simulink model "MPC_framework"  (Simulink 6.4)
settings: Solver=FixedStepDiscrete  StartTime=0.0  StopTime=10.0  FixedStep=0.01  RelTol=1e-3
PreLoadFcn:
  | RTWConfigurationCB('preloadfcn', bdroot);
InitFcn:
  | % START RTW CONFIGURATION CODE %
  | RTWConfigurationCB('rtw_target_initfcn',gcs);
  | % END RTW CONFIGURATION CODE %
undefined symbols (not defined in the file): a1, a2, DA_max_saturation, DA_min_saturation, DiscIntNeverNeededParam, fundamental_sample_time, incntr_half_val, init_1_message, init_2_message, init_ack_async_message, init_ack_sync_message, motor_negative_value_seg_1, motor_negative_value_seg_2, motor_positive_value_seg_1, motor_positive_value_seg_2, motor_stopped_value, ticks_per_trajectory_time, trajectory_time
libraries: canblocks x16, mpc555toucan x16, simulink x8, mpc555drivers x1
(part 1 of 2)
CloseFcn:
  | rtwprivate ssgencode ModelCloseRequest MPC_framework
settings Model: LastModifiedBy=Developer  ProdHWDeviceType=Motorola PowerPC
settings OptimizationCC: OptimizeModelRefInitCode=on  LifeSpan=1
settings HardwareCC: ProdIntDivRoundTo=Zero  ProdEndianess=BigEndian  ProdHWDeviceType=Motorola PowerPC
settings RTWCC: SystemTargetFile=mpc555rt.tlc  TemplateMakefile=mpc555rt.tmf  Description=Embedded Target for Motorola MPC555 (real-time target)  ProcessScript=mpc555rt_make_rtw_hook
settings CodeAppCC: IgnoreCustomStorageClasses=off
settings STFCustomTargetCC: TargetFcnLib=codewarrior_tfl_tmw.mat  TargetLibSuffix=.a  TargetPreCompLibLocation=C:\MATLAB\R2006a\toolbox\rtw\targets\mpc555dk\drivers\lib\CODE_WARRIOR  GenFloatMathFcnCalls=ISO_C  CombineOutputUpdateFcns=on  IncludeERTFirstTime=on  ERTCustomFileBanners=on  SupportContinuousTime=off  SupportNonInlinedSFcns=off  SystemTargetFile=mpc555rt.tlc
settings ERTTargetCC: TargetFcnLib=codewarrior_tfl_tmw.mat  TargetPreCompLibLocation=C:\MATLAB\R2006a\toolbox\rtw\targets\mpc555dk\drivers\lib\CODE_WARRIOR  GenFloatMathFcnCalls=ISO_C  IncludeERTFirstTime=on  ERTFirstTimeCompliant=off  InlinedParameterPlacement=NonHierarchical  ERTCustomFileTemplate=example_file_process.tlc  InitialValueSource=Model
settings CustomProperty: DataType=RTWOptions_EnumType__toolbox_rtw_targets_mpc555dk_mpc555dk_mpc555rt_MPC555_OPTIMIZATION_SWITCH  Value=speed
settings EnumStrPairs: String=speed

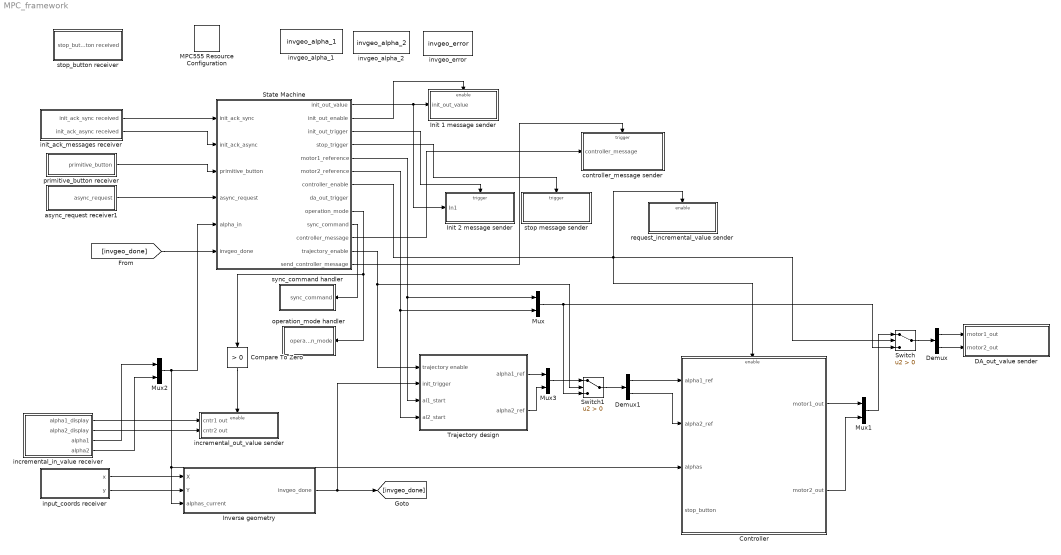
== system MPC_framework ==
  Compare To Zero : simulink/Logic and Bit Operations/Compare To Zero  Orientation=down  SystemSampleTime=-1  relop=>  LogicOutDataTypeMode=uint8  ZeroCross=off
  Controller : Subsystem
  DA_out_value sender : Subsystem  TreatAsAtomicUnit=on
  Demux : Demux  Outputs=2
  Demux1 : Demux  Outputs=2
  Init 1 message sender : Subsystem  TreatAsAtomicUnit=on
  Init 2 message sender : Subsystem  TreatAsAtomicUnit=on
  Inverse geometry : Subsystem  TreatAsAtomicUnit=on
  MPC555 Resource Configuration : mpc555drivers/MPC555 Resource Configuration  Tag=RTW CONFIGURATION BLOCK  Priority=-100000  SystemSampleTime=-1  oldParentName=MPC_framework  oldBlockName=|
      | MPC_framework/MPC555
      | Resource
      | Configuration
  Mux{,1..3} (4 alike) : Mux  Inputs=2
  State Machine : Stateflow chart
  Switch : Switch  Criteria=u2 > Threshold  SampleTime=fundamental_sample_time  InputSameDT=on
  Switch1 : Switch  Criteria=u2 > Threshold  SampleTime=fundamental_sample_time  InputSameDT=on
  Trajectory design : Subsystem
  async_request receiver1 : Subsystem
  controller_message sender : Subsystem  TreatAsAtomicUnit=on
  incremental_in_value receiver : Subsystem
  incremental_out_value sender : Subsystem  TreatAsAtomicUnit=on
  init_ack_messages receiver : Subsystem
  input_coords receiver : Subsystem
  invgeo_alpha_1 : DataStoreMemory  DataStoreName=invgeo_alpha_1  ReadBeforeWriteMsg=error  WriteAfterWriteMsg=error  WriteAfterReadMsg=error  InitialValue=0  DataType=single
  invgeo_alpha_2 : DataStoreMemory  DataStoreName=invgeo_alpha_2  ReadBeforeWriteMsg=error  WriteAfterWriteMsg=error  WriteAfterReadMsg=error  InitialValue=0  DataType=single
  invgeo_error : DataStoreMemory  DataStoreName=invgeo_error  ReadBeforeWriteMsg=error  WriteAfterWriteMsg=error  WriteAfterReadMsg=error  InitialValue=255  DataType=uint8
  operation_mode handler : Subsystem  Orientation=left
  primitive_button receiver : Subsystem
  request_incremental_value sender : Subsystem  TreatAsAtomicUnit=on
  stop message sender : Subsystem  TreatAsAtomicUnit=on
  stop_button receiver : Subsystem
  sync_command handler : Subsystem  Orientation=left
  wires:
  State Machine/1(init_out_value) -> Init 2 message sender/1(In1), Init 1 message sender/1(init_out_value)
  State Machine/2(init_out_enable) -> Init 1 message sender/Enable
  init_ack_messages receiver/1(init_ack_sync received) -> State Machine/1(init_ack_sync)
  init_ack_messages receiver/2(init_ack_async received) -> State Machine/2(init_ack_async)
  State Machine/3(init_out_trigger) -> Init 2 message sender/Trigger
  State Machine/4(stop_trigger) -> stop message sender/Trigger
  primitive_button receiver/1(primitive_button) -> State Machine/3(primitive_button)
  State Machine/7(controller_enable) -> Controller/Enable, Switch/2, request_incremental_value sender/Enable
  State Machine/5(motor1_reference) -> Mux/1, Trajectory design/3(al1_start)
  Controller/1(motor1_out) -> Mux1/1
  Controller/2(motor2_out) -> Mux1/2
  Mux1/1 -> Switch/1
  Mux/1 -> Switch/3, Switch1/3
  Switch/1 -> Demux/1
  Demux/1 -> DA_out_value sender/1(motor1_out)
  Demux/2 -> DA_out_value sender/2(motor2_out)
  State Machine/9(operation_mode) -> Compare To Zero/1, operation_mode handler/1(operation_mode)
  async_request receiver1/1(async_request) -> State Machine/4(async_request)
  State Machine/10(sync_command) -> sync_command handler/1(sync_command)
  Mux2/1 -> State Machine/5(alpha_in), Inverse geometry/3(alphas_current), Controller/3(alphas)
  State Machine/11(controller_message) -> controller_message sender/1(controller_message)
  State Machine/13(send_controller_message) -> controller_message sender/Trigger
  input_coords receiver/1(x) -> Inverse geometry/1(X)
  input_coords receiver/2(y) -> Inverse geometry/2(Y)
  Inverse geometry/1(invgeo_done) -> [invgeo_done], Trajectory design/2(init_trigger)
  [invgeo_done] -> State Machine/6(invgeo_done)
  State Machine/6(motor2_reference) -> Mux/2, Trajectory design/4(al2_start)
  Trajectory design/1(alpha1_ref) -> Mux3/1
  Trajectory design/2(alpha2_ref) -> Mux3/2
  Mux3/1 -> Switch1/1
  State Machine/12(trajectory_enable) -> Trajectory design/1(trajectory enable), Switch1/2
  Switch1/1 -> Demux1/1
  Demux1/1 -> Controller/1(alpha1_ref)
  Demux1/2 -> Controller/2(alpha2_ref)
  incremental_in_value receiver/3(alpha1) -> Mux2/1
  incremental_in_value receiver/4(alpha2) -> Mux2/2
  Compare To Zero/1 -> incremental_out_value sender/Enable
  incremental_in_value receiver/1(alpha1_display) -> incremental_out_value sender/1(cntr1 out)
  incremental_in_value receiver/2(alpha2_display) -> incremental_out_value sender/2(cntr2 out)

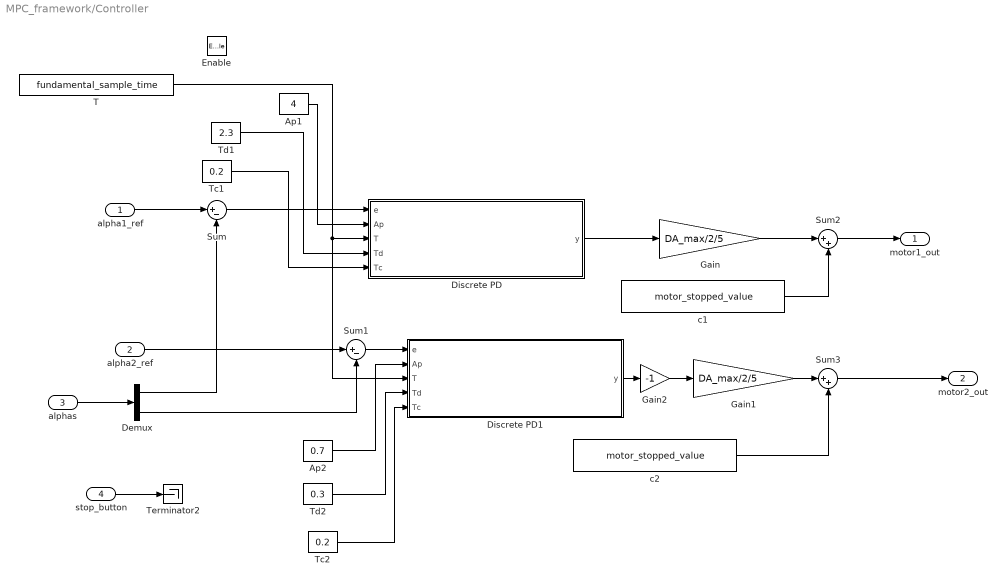
== system MPC_framework/Controller ==
  alpha1_ref : Inport
  alpha2_ref : Inport  Port=2
  alphas : Inport  Port=3
  stop_button : Inport  Port=4
  Enable : EnablePort  StatesWhenEnabling=reset
  Ap1 : Constant  Value=4  OutDataTypeMode=single  OutDataType=sfix(16)  ConRadixGroup=Use specified scaling  OutScaling=2^0  SampleTime=inf  FramePeriod=inf
  Ap2 : Constant  Value=0.7  OutDataTypeMode=single  OutDataType=sfix(16)  ConRadixGroup=Use specified scaling  OutScaling=2^0  SampleTime=inf  FramePeriod=inf
  Demux : Demux  Outputs=2
  Discrete PD : Subsystem
  Discrete PD1 : Subsystem
  Gain : Gain  Gain=DA_max/2/5  ParameterDataTypeMode=Specify via dialog  ParameterDataType=float('single')  OutDataTypeMode=Specify via dialog  OutDataType=float('single')
  Gain1 : Gain  Gain=DA_max/2/5  ParameterDataTypeMode=Specify via dialog  ParameterDataType=float('single')  OutDataTypeMode=Specify via dialog  OutDataType=float('single')
  Gain2 : Gain  Gain=-1  ParameterDataTypeMode=Specify via dialog  ParameterDataType=float('single')  OutDataTypeMode=Specify via dialog  OutDataType=float('single')
  Sum : Sum  Inputs=|+-
  Sum1 : Sum  Inputs=|+-
  Sum2 : Sum  Inputs=|++  InputSameDT=on
  Sum3 : Sum  Inputs=|++  InputSameDT=on
  T : Constant  Value=fundamental_sample_time  OutDataTypeMode=single  OutDataType=sfix(16)  ConRadixGroup=Use specified scaling  OutScaling=2^0  SampleTime=inf  FramePeriod=inf
  Tc1 : Constant  Value=0.2  OutDataTypeMode=single  OutDataType=sfix(16)  ConRadixGroup=Use specified scaling  OutScaling=2^0  SampleTime=inf  FramePeriod=inf
  Tc2 : Constant  Value=0.2  OutDataTypeMode=single  OutDataType=sfix(16)  ConRadixGroup=Use specified scaling  OutScaling=2^0  SampleTime=inf  FramePeriod=inf
  Td1 : Constant  Value=2.3  OutDataTypeMode=single  OutDataType=sfix(16)  ConRadixGroup=Use specified scaling  OutScaling=2^0  SampleTime=inf  FramePeriod=inf
  Td2 : Constant  Value=0.3  OutDataTypeMode=single  OutDataType=sfix(16)  ConRadixGroup=Use specified scaling  OutScaling=2^0  SampleTime=inf  FramePeriod=inf
  Terminator2 : Terminator
  c1 : Constant  Value=motor_stopped_value  OutDataTypeMode=single  OutDataType=sfix(16)  ConRadixGroup=Use specified scaling  OutScaling=2^0  SampleTime=inf  FramePeriod=inf
  c2 : Constant  Value=motor_stopped_value  OutDataTypeMode=single  OutDataType=sfix(16)  ConRadixGroup=Use specified scaling  OutScaling=2^0  SampleTime=inf  FramePeriod=inf
  motor1_out : Outport
  motor2_out : Outport  Port=2
  wires:
  stop_button/1 -> Terminator2/1
  alphas/1 -> Demux/1
  alpha1_ref/1 -> Sum/1
  Sum/1 -> Discrete PD/1(e)
  Ap1/1 -> Discrete PD/2(Ap)
  T/1 -> Discrete PD/3(T), Discrete PD1/3(T)
  Td1/1 -> Discrete PD/4(Td)
  Tc1/1 -> Discrete PD/5(Tc)
  Demux/1 -> Sum/2
  Sum1/1 -> Discrete PD1/1(e)
  alpha2_ref/1 -> Sum1/1
  Demux/2 -> Sum1/2
  Ap2/1 -> Discrete PD1/2(Ap)
  Td2/1 -> Discrete PD1/4(Td)
  Tc2/1 -> Discrete PD1/5(Tc)
  Discrete PD1/1(y) -> Gain2/1
  c1/1 -> Sum2/2
  Gain/1 -> Sum2/1
  Discrete PD/1(y) -> Gain/1
  Sum2/1 -> motor1_out/1
  c2/1 -> Sum3/2
  Gain1/1 -> Sum3/1
  Gain2/1 -> Gain1/1
  Sum3/1 -> motor2_out/1

== system MPC_framework/DA_out_value sender ==
  motor1_out : Inport
  motor2_out : Inport  Port=2
  Constant : Constant  Value=motor_stopped_value  OutDataType=sfix(16)  ConRadixGroup=Use specified scaling  OutScaling=2^0  SampleTime=inf  FramePeriod=inf
  DA_out_value message packing : canblocks/CAN Message Packing (CANdb)
  Saturation : Saturate  UpperLimit=DA_max_saturation  LowerLimit=DA_min_saturation
  Saturation1 : Saturate  UpperLimit=DA_max_saturation  LowerLimit=DA_min_saturation
  Saturation2 : Saturate  UpperLimit=DA_max_saturation  LowerLimit=DA_min_saturation
  TouCAN Transmit : mpc555toucan/TouCAN Transmit  SystemSampleTime=-1  module=A  tx_mode=Queued transmission with shared buffer  fifo_queue_length=8  bufferids=0  buffers_used=0, 1, 2  t=fundamental_sample_time  enablePassThru=off
  wires:
  DA_out_value message packing/1 -> TouCAN Transmit/1
  motor1_out/1 -> Saturation2/1
  motor2_out/1 -> Saturation1/1
  Constant/1 -> Saturation/1
  Saturation/1 -> DA_out_value message packing/1
  Saturation1/1 -> DA_out_value message packing/2
  Saturation2/1 -> DA_out_value message packing/3

== system MPC_framework/Init 1 message sender ==
  init_out_value : Inport
  Enable : EnablePort
  TouCAN Transmit : mpc555toucan/TouCAN Transmit  SystemSampleTime=-1  module=A  tx_mode=Queued transmission with shared buffer  fifo_queue_length=8  bufferids=0  buffers_used=0, 1, 2  t=init_1_message_frequency  enablePassThru=off
  init message packing : canblocks/CAN Message Packing (CANdb)
  wires:
  init_out_value/1 -> init message packing/1
  init message packing/1 -> TouCAN Transmit/1

== system MPC_framework/Init 2 message sender ==
  In1 : Inport
  Trigger : TriggerPort
  TouCAN Transmit : mpc555toucan/TouCAN Transmit  SystemSampleTime=-1  module=A  tx_mode=Queued transmission with shared buffer  fifo_queue_length=8  bufferids=0  buffers_used=0, 1, 2  t=-1  enablePassThru=off
  init message packing : canblocks/CAN Message Packing (CANdb)
  wires:
  In1/1 -> init message packing/1
  init message packing/1 -> TouCAN Transmit/1

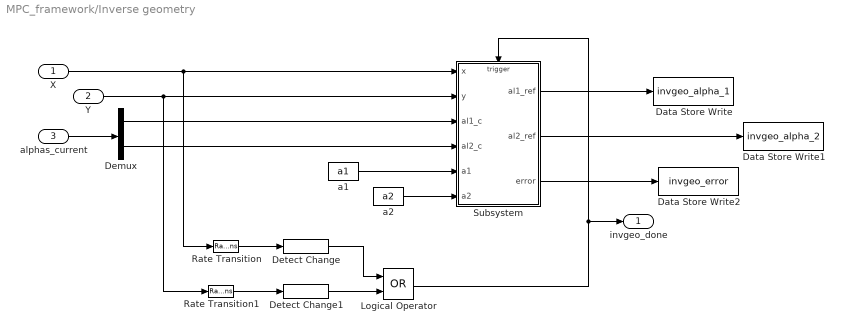
== system MPC_framework/Inverse geometry ==
  X : Inport
  Y : Inport  Port=2
  alphas_current : Inport  Port=3
  Data Store Write : DataStoreWrite  DataStoreName=invgeo_alpha_1  SampleTime=fundamental_sample_time
  Data Store Write1 : DataStoreWrite  DataStoreName=invgeo_alpha_2  SampleTime=fundamental_sample_time
  Data Store Write2 : DataStoreWrite  DataStoreName=invgeo_error  SampleTime=fundamental_sample_time
  Demux : Demux  Outputs=2
  Detect Change : simulink/Logic and Bit Operations/Detect Change  SystemSampleTime=-1  vinit=0
  Detect Change1 : simulink/Logic and Bit Operations/Detect Change  SystemSampleTime=-1  vinit=0
  Logical Operator : Logic  Operator=OR  AllPortsSameDT=off  OutDataTypeMode=Specify via dialog
  Rate Transition : RateTransition  OutPortSampleTime=fundamental_sample_time
  Rate Transition1 : RateTransition  OutPortSampleTime=fundamental_sample_time
  Subsystem : Subsystem
  a1 : Constant  Value=a1  OutDataTypeMode=single  OutDataType=sfix(16)  ConRadixGroup=Use specified scaling  OutScaling=2^0  SampleTime=inf  FramePeriod=inf
  a2 : Constant  Value=a2  OutDataTypeMode=single  OutDataType=sfix(16)  ConRadixGroup=Use specified scaling  OutScaling=2^0  SampleTime=inf  FramePeriod=inf
  invgeo_done : Outport
  wires:
  X/1 -> Rate Transition/1, Subsystem/1(x)
  Y/1 -> Rate Transition1/1, Subsystem/2(y)
  alphas_current/1 -> Demux/1
  Demux/1 -> Subsystem/3(al1_c)
  Demux/2 -> Subsystem/4(al2_c)
  a1/1 -> Subsystem/5(a1)
  a2/1 -> Subsystem/6(a2)
  Subsystem/1(al1_ref) -> Data Store Write/1
  Subsystem/2(al2_ref) -> Data Store Write1/1
  Subsystem/3(error) -> Data Store Write2/1
  Rate Transition/1 -> Detect Change/1
  Detect Change/1 -> Logical Operator/1
  Detect Change1/1 -> Logical Operator/2
  Rate Transition1/1 -> Detect Change1/1
  Logical Operator/1 -> invgeo_done/1, Subsystem/Trigger

== system MPC_framework/Trajectory design ==
  trajectory enable : Inport
  init_trigger : Inport  Port=2
  al1_start : Inport  Port=3
  al2_start : Inport  Port=4
  Data Store Read : DataStoreRead  DataStoreName=invgeo_alpha_1  SampleTime=fundamental_sample_time
  Data Store Read1 : DataStoreRead  DataStoreName=invgeo_alpha_2  SampleTime=fundamental_sample_time
  Trajectory design1 : Subsystem
  alpha1_ref : Outport
  alpha2_ref : Outport  Port=2
  wires:
  trajectory enable/1 -> Trajectory design1/1(trajectory enable)
  init_trigger/1 -> Trajectory design1/2(init trigger)
  al1_start/1 -> Trajectory design1/3(al1_start)
  Data Store Read/1 -> Trajectory design1/4(al1_end)
  al2_start/1 -> Trajectory design1/5(al2_start)
  Data Store Read1/1 -> Trajectory design1/6(al2_end)
  Trajectory design1/1(al1) -> alpha1_ref/1
  Trajectory design1/4(al2) -> alpha2_ref/1

== system MPC_framework/async_request receiver1 ==
  async_request message receive : mpc555toucan/TouCAN Receive  SystemSampleTime=-1  module=A  ids=hex2dec('0C')  notification_type=Function Call Outport  auto_select_buffer=on  bufferids=3  use_queue=off  queue_length=3  message_type=Standard (11-bit identifier)  t=-1
  async_request message unpacking : Subsystem  TreatAsAtomicUnit=on
      settings: OpenFcn=open_system(gcb, 'force');
      mask Type: CAN Message Unpacking (CANdb)
      mask Description: CAN Message Unpacking (CANdb) Function-Call Subsystem Template
      mask Help: helpview([docroot '/toolbox/can_blocks/can_blocks.map'], 'template_CANdb_msg_unpack');
  async_request : Outport
  wires:
  async_request message receive/1 -> async_request message unpacking/Trigger
  async_request message receive/2 -> async_request message unpacking/1(Msg)
  async_request message unpacking/1(async_request) -> async_request/1

== system MPC_framework/controller_message sender ==
  controller_message : Inport
  function : TriggerPort  TriggerType=function-call
  TouCAN Transmit : mpc555toucan/TouCAN Transmit  SystemSampleTime=-1  module=A  tx_mode=Queued transmission with shared buffer  fifo_queue_length=8  bufferids=0  buffers_used=0, 1, 2  t=-1  enablePassThru=off
  controller_message packing : canblocks/CAN Message Packing (CANdb)
  wires:
  controller_message packing/1 -> TouCAN Transmit/1
  controller_message/1 -> controller_message packing/1

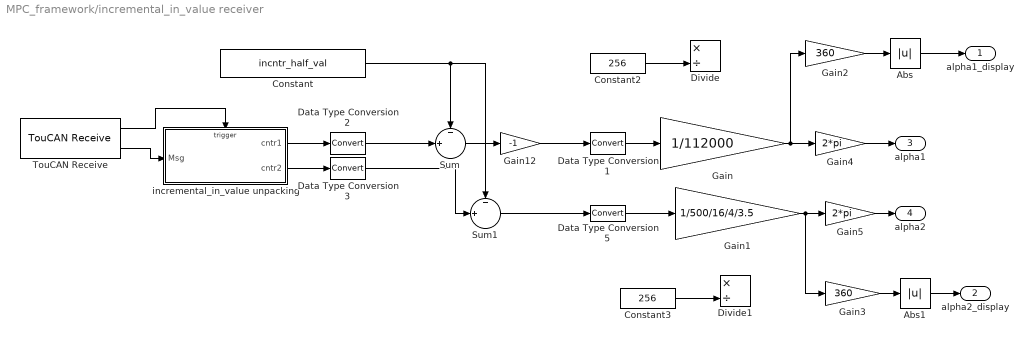
== system MPC_framework/incremental_in_value receiver ==
  Abs : Abs  SampleTime=-1  SaturateOnIntegerOverflow=off
  Abs1 : Abs  SampleTime=-1  SaturateOnIntegerOverflow=off
  Constant : Constant  Value=incntr_half_val  OutDataTypeMode=int32  OutDataType=sfix(16)  ConRadixGroup=Use specified scaling  OutScaling=2^0  SampleTime=inf  FramePeriod=inf
  Constant2 : Constant  Value=256  OutDataTypeMode=int32  OutDataType=sfix(16)  ConRadixGroup=Use specified scaling  OutScaling=2^0  SampleTime=inf  FramePeriod=inf
  Constant3 : Constant  Value=256  OutDataTypeMode=int32  OutDataType=sfix(16)  ConRadixGroup=Use specified scaling  OutScaling=2^0  SampleTime=inf  FramePeriod=inf
  Data Type Conversion1 : DataTypeConversion  OutDataTypeMode=single
  Data Type Conversion2 : DataTypeConversion  OutDataTypeMode=int32
  Data Type Conversion3 : DataTypeConversion  OutDataTypeMode=int32
  Data Type Conversion5 : DataTypeConversion  OutDataTypeMode=single
  Divide : Product  Inputs=*/  OutDataTypeMode=int32  OutScaling=2^-10  InputSameDT=on
  Divide1 : Product  Inputs=*/  OutDataTypeMode=int32  OutScaling=2^-10  InputSameDT=on
  Gain : Gain  Gain=1/112000  ParameterDataTypeMode=Specify via dialog  ParameterDataType=float('single')  OutDataTypeMode=Specify via dialog  OutDataType=float('single')
  Gain1 : Gain  Gain=1/500/16/4/3.5  SaturateOnIntegerOverflow=on
  Gain12 : Gain  Gain=-1  SaturateOnIntegerOverflow=on
  Gain2 : Gain  Gain=360  ParameterDataTypeMode=Specify via dialog  ParameterDataType=float('single')  OutDataTypeMode=Specify via dialog  OutDataType=float('single')
  Gain3 : Gain  Gain=360  ParameterDataTypeMode=Specify via dialog  ParameterDataType=float('single')  OutDataTypeMode=Specify via dialog  OutDataType=float('single')
  Gain4 : Gain  Gain=2*pi  ParameterDataTypeMode=Specify via dialog  ParameterDataType=float('single')  OutDataTypeMode=Specify via dialog  OutDataType=float('single')
  Gain5 : Gain  Gain=2*pi  ParameterDataTypeMode=Specify via dialog  ParameterDataType=float('single')  OutDataTypeMode=Specify via dialog  OutDataType=float('single')
  Sum : Sum  Inputs=-|+||  OutDataTypeMode=int32  InputSameDT=on
  Sum1 : Sum  Inputs=-|+||  OutDataTypeMode=int32  InputSameDT=on
  TouCAN Receive : mpc555toucan/TouCAN Receive  SystemSampleTime=-1  module=A  ids=hex2dec('07')  notification_type=Function Call Outport  auto_select_buffer=on  bufferids=4  use_queue=off  queue_length=3  message_type=Standard (11-bit identifier)  t=-1
  incremental_in_value unpacking : Subsystem  TreatAsAtomicUnit=on
      settings: OpenFcn=open_system(gcb, 'force');
      mask Type: CAN Message Unpacking (CANdb)
      mask Description: CAN Message Unpacking (CANdb) Function-Call Subsystem Template
      mask Help: helpview([docroot '/toolbox/can_blocks/can_blocks.map'], 'template_CANdb_msg_unpack');
  alpha1_display : Outport
  alpha2_display : Outport  Port=2
  alpha1 : Outport  Port=3
  alpha2 : Outport  Port=4
  wires:
  TouCAN Receive/2 -> incremental_in_value unpacking/1(Msg)
  TouCAN Receive/1 -> incremental_in_value unpacking/Trigger
  Sum/1 -> Gain12/1
  Sum1/1 -> Data Type Conversion5/1
  Constant/1 -> Sum1/1, Sum/1
  Data Type Conversion3/1 -> Sum1/2
  Data Type Conversion5/1 -> Gain1/1
  Constant2/1 -> Divide/2
  Constant3/1 -> Divide1/2
  Gain/1 -> Gain2/1, Gain4/1
  Gain1/1 -> Gain3/1, Gain5/1
  Data Type Conversion1/1 -> Gain/1
  incremental_in_value unpacking/1(cntr1) -> Data Type Conversion2/1
  Data Type Conversion2/1 -> Sum/2
  incremental_in_value unpacking/2(cntr2) -> Data Type Conversion3/1
  Gain4/1 -> alpha1/1
  Gain5/1 -> alpha2/1
  Gain12/1 -> Data Type Conversion1/1
  Gain2/1 -> Abs/1
  Gain3/1 -> Abs1/1
  Abs/1 -> alpha1_display/1
  Abs1/1 -> alpha2_display/1

== system MPC_framework/incremental_out_value sender ==
  cntr1 out : Inport
  cntr2 out : Inport  Port=2
  Enable : EnablePort
  Data Type Conversion : DataTypeConversion  OutDataTypeMode=uint16
  Data Type Conversion1 : DataTypeConversion  OutDataTypeMode=uint16
  TouCAN Transmit : mpc555toucan/TouCAN Transmit  SystemSampleTime=-1  module=A  tx_mode=Queued transmission with shared buffer  fifo_queue_length=8  bufferids=0  buffers_used=0, 1, 2  t=-1  enablePassThru=off
  incremental_out_value message packing : canblocks/CAN Message Packing (CANdb)
  wires:
  incremental_out_value message packing/1 -> TouCAN Transmit/1
  cntr1 out/1 -> Data Type Conversion/1
  cntr2 out/1 -> Data Type Conversion1/1
  Data Type Conversion/1 -> incremental_out_value message packing/1
  Data Type Conversion1/1 -> incremental_out_value message packing/2

== system MPC_framework/init_ack_messages receiver ==
  CAN Message Unpacking (CANdb) : Subsystem  TreatAsAtomicUnit=on
      settings: OpenFcn=open_system(gcb, 'force');
      mask Type: CAN Message Unpacking (CANdb)
      mask Description: CAN Message Unpacking (CANdb) Function-Call Subsystem Template
      mask Help: helpview([docroot '/toolbox/can_blocks/can_blocks.map'], 'template_CANdb_msg_unpack');
  CAN Message Unpacking (CANdb)1 : Subsystem  TreatAsAtomicUnit=on
      settings: OpenFcn=open_system(gcb, 'force');
      mask Type: CAN Message Unpacking (CANdb)
      mask Description: CAN Message Unpacking (CANdb) Function-Call Subsystem Template
      mask Help: helpview([docroot '/toolbox/can_blocks/can_blocks.map'], 'template_CANdb_msg_unpack');
  TouCAN Receive : mpc555toucan/TouCAN Receive  SystemSampleTime=-1  module=A  ids=hex2dec('02')  notification_type=Function Call Outport  auto_select_buffer=on  bufferids=5  use_queue=off  queue_length=3  message_type=Standard (11-bit identifier)  t=-1
  TouCAN Receive1 : mpc555toucan/TouCAN Receive  SystemSampleTime=-1  module=A  ids=hex2dec('03')  notification_type=Function Call Outport  auto_select_buffer=on  bufferids=6  use_queue=off  queue_length=3  message_type=Standard (11-bit identifier)  t=-1
  init_ack_sync received : Outport
  init_ack_async received : Outport  Port=2
  wires:
  TouCAN Receive/1 -> CAN Message Unpacking (CANdb)/Trigger
  TouCAN Receive/2 -> CAN Message Unpacking (CANdb)/1(Msg)
  CAN Message Unpacking (CANdb)/1(init_ack_sync received) -> init_ack_sync received/1
  TouCAN Receive1/1 -> CAN Message Unpacking (CANdb)1/Trigger
  TouCAN Receive1/2 -> CAN Message Unpacking (CANdb)1/1(Msg)
  CAN Message Unpacking (CANdb)1/1(init_ack_async received) -> init_ack_async received/1

== system MPC_framework/input_coords receiver ==
  input_coords message receive : mpc555toucan/TouCAN Receive  SystemSampleTime=-1  module=A  ids=hex2dec('0F')  notification_type=Function Call Outport  auto_select_buffer=on  bufferids=7  use_queue=off  queue_length=3  message_type=Standard (11-bit identifier)  t=-1
  input_coords message unpacking : Subsystem  TreatAsAtomicUnit=on
      settings: OpenFcn=open_system(gcb, 'force');
      mask Type: CAN Message Unpacking (CANdb)
      mask Description: CAN Message Unpacking (CANdb) Function-Call Subsystem Template
      mask Help: helpview([docroot '/toolbox/can_blocks/can_blocks.map'], 'template_CANdb_msg_unpack');
  x : Outport
  y : Outport  Port=2
  wires:
  input_coords message unpacking/1(x) -> x/1
  input_coords message unpacking/2(y) -> y/1
  input_coords message receive/2 -> input_coords message unpacking/1(Msg)
  input_coords message receive/1 -> input_coords message unpacking/Trigger

== system MPC_framework/operation_mode handler ==
  operation_mode : Inport
  Detect Change : simulink/Logic and Bit Operations/Detect Change  SystemSampleTime=-1  vinit=0
  operation_mode_changed sender : Subsystem  TreatAsAtomicUnit=on
  wires:
  Detect Change/1 -> operation_mode_changed sender/Trigger
  operation_mode/1 -> operation_mode_changed sender/1(operation_mode), Detect Change/1

== system MPC_framework/primitive_button receiver ==
  primitive_button message receive : mpc555toucan/TouCAN Receive  SystemSampleTime=-1  module=A  ids=hex2dec('08')  notification_type=Function Call Outport  auto_select_buffer=on  bufferids=8  use_queue=off  queue_length=3  message_type=Standard (11-bit identifier)  t=-1
  primitive_button message unpacking : Subsystem  TreatAsAtomicUnit=on
      settings: OpenFcn=open_system(gcb, 'force');
      mask Type: CAN Message Unpacking (CANdb)
      mask Description: CAN Message Unpacking (CANdb) Function-Call Subsystem Template
      mask Help: helpview([docroot '/toolbox/can_blocks/can_blocks.map'], 'template_CANdb_msg_unpack');
  primitive_button : Outport
  wires:
  primitive_button message unpacking/1("primitive_button ") -> primitive_button/1
  primitive_button message receive/2 -> primitive_button message unpacking/1(Msg)
  primitive_button message receive/1 -> primitive_button message unpacking/Trigger

== system MPC_framework/request_incremental_value sender ==
  Enable : EnablePort
  Constant : Constant  Value=1  OutDataTypeMode=uint8  OutDataType=sfix(16)  ConRadixGroup=Use specified scaling  OutScaling=2^0  SampleTime=0.1  FramePeriod=inf
  TouCAN Transmit : mpc555toucan/TouCAN Transmit  SystemSampleTime=-1  module=A  tx_mode=Queued transmission with shared buffer  fifo_queue_length=8  bufferids=0  buffers_used=0, 1, 2  t=-1  enablePassThru=off
  request_incremental_value message packing : canblocks/CAN Message Packing (CANdb)
  wires:
  Constant/1 -> request_incremental_value message packing/1
  request_incremental_value message packing/1 -> TouCAN Transmit/1

== system MPC_framework/stop message sender ==
  Trigger : TriggerPort
  Constant : Constant  Value=1  OutDataTypeMode=uint8  OutDataType=sfix(16)  ConRadixGroup=Use specified scaling  OutScaling=2^0  SampleTime=inf  FramePeriod=inf
  TouCAN Transmit : mpc555toucan/TouCAN Transmit  SystemSampleTime=-1  module=A  tx_mode=Queued transmission with shared buffer  fifo_queue_length=8  bufferids=0  buffers_used=0, 1, 2  t=-1  enablePassThru=off
  stop message packing : canblocks/CAN Message Packing (CANdb)
  wires:
  stop message packing/1 -> TouCAN Transmit/1
  Constant/1 -> stop message packing/1

== system MPC_framework/stop_button receiver ==
  TouCAN Receive : mpc555toucan/TouCAN Receive  SystemSampleTime=-1  module=A  ids=hex2dec('04')  notification_type=Function Call Outport  auto_select_buffer=on  bufferids=9  use_queue=off  queue_length=3  message_type=Standard (11-bit identifier)  t=-1
  stop_button message packing : Subsystem  TreatAsAtomicUnit=on
      settings: OpenFcn=open_system(gcb, 'force');
      mask Type: CAN Message Unpacking (CANdb)
      mask Description: CAN Message Unpacking (CANdb) Function-Call Subsystem Template
      mask Help: helpview([docroot '/toolbox/can_blocks/can_blocks.map'], 'template_CANdb_msg_unpack');
  stop_button received : Outport
  wires:
  TouCAN Receive/1 -> stop_button message packing/Trigger
  TouCAN Receive/2 -> stop_button message packing/1(Msg)
  stop_button message packing/1(stop_button received) -> stop_button received/1

== system MPC_framework/sync_command handler ==
  sync_command : Inport
  Compare To Zero1 : simulink/Logic and Bit Operations/Compare To Zero  SystemSampleTime=-1  relop=>  LogicOutDataTypeMode=uint8  ZeroCross=off
  Detect Change2 : simulink/Logic and Bit Operations/Detect Change  SystemSampleTime=-1  vinit=0
  Logical Operator : Logic  AllPortsSameDT=off  OutDataTypeMode=Boolean
  sync_command sender : Subsystem  TreatAsAtomicUnit=on
  wires:
  Detect Change2/1 -> Logical Operator/1
  Compare To Zero1/1 -> Logical Operator/2
  Logical Operator/1 -> sync_command sender/Trigger
  sync_command/1 -> Detect Change2/1, Compare To Zero1/1, sync_command sender/1(sync_command)

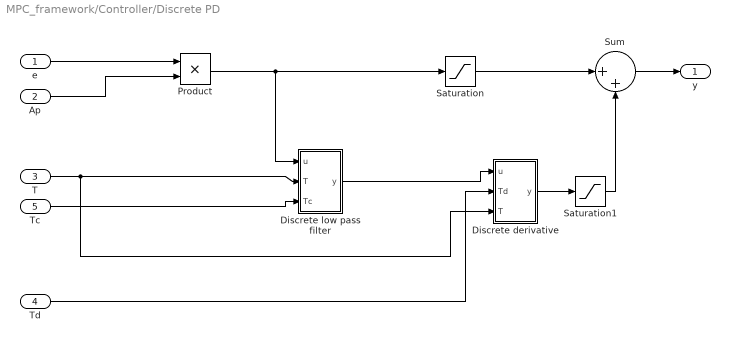
== system MPC_framework/Controller/Discrete PD ==
  e : Inport  OutDataType=fixdt(1,16,0)  OutScaling=[]
  Ap : Inport  Port=2  OutDataType=fixdt(1,16,0)  OutScaling=[]
  T : Inport  Port=3  OutDataType=fixdt(1,16,0)  OutScaling=[]
  Td : Inport  Port=4  OutDataType=fixdt(1,16,0)  OutScaling=[]
  Tc : Inport  Port=5  OutDataType=fixdt(1,16,0)  OutScaling=[]
  Discrete derivative : Subsystem
  Discrete low pass filter : Subsystem
  Product : Product  OutDataTypeMode=single  OutDataType=fixdt(1,16,0)  OutScaling=[]  RndMeth=Zero  InputSameDT=on
  Saturation : Saturate
  Saturation1 : Saturate
  Sum : Sum  Inputs=|++  OutDataType=fixdt(1,16,0)  OutScaling=[]
  y : Outport  OutDataType=fixdt(1,16,0)  OutScaling=[]
  wires:
  Product/1 -> Discrete low pass filter/1(u), Saturation/1
  e/1 -> Product/1
  Sum/1 -> y/1
  Ap/1 -> Product/2
  T/1 -> Discrete low pass filter/2(T), Discrete derivative/3(T)
  Tc/1 -> Discrete low pass filter/3(Tc)
  Td/1 -> Discrete derivative/2(Td)
  Discrete derivative/1(y) -> Saturation1/1
  Discrete low pass filter/1(y) -> Discrete derivative/1(u)
  Saturation/1 -> Sum/1
  Saturation1/1 -> Sum/2

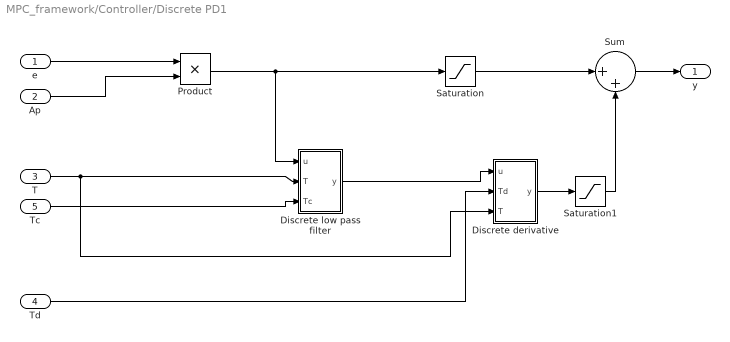
== system MPC_framework/Controller/Discrete PD1 ==
  e : Inport  OutDataType=fixdt(1,16,0)  OutScaling=[]
  Ap : Inport  Port=2  OutDataType=fixdt(1,16,0)  OutScaling=[]
  T : Inport  Port=3  OutDataType=fixdt(1,16,0)  OutScaling=[]
  Td : Inport  Port=4  OutDataType=fixdt(1,16,0)  OutScaling=[]
  Tc : Inport  Port=5  OutDataType=fixdt(1,16,0)  OutScaling=[]
  Discrete derivative : Subsystem
  Discrete low pass filter : Subsystem
  Product : Product  OutDataTypeMode=single  OutDataType=fixdt(1,16,0)  OutScaling=[]  RndMeth=Zero  InputSameDT=on
  Saturation : Saturate
  Saturation1 : Saturate
  Sum : Sum  Inputs=|++  OutDataType=fixdt(1,16,0)  OutScaling=[]
  y : Outport  OutDataType=fixdt(1,16,0)  OutScaling=[]
  wires:
  Product/1 -> Discrete low pass filter/1(u), Saturation/1
  e/1 -> Product/1
  Sum/1 -> y/1
  Ap/1 -> Product/2
  T/1 -> Discrete low pass filter/2(T), Discrete derivative/3(T)
  Tc/1 -> Discrete low pass filter/3(Tc)
  Td/1 -> Discrete derivative/2(Td)
  Discrete derivative/1(y) -> Saturation1/1
  Discrete low pass filter/1(y) -> Discrete derivative/1(u)
  Saturation/1 -> Sum/1
  Saturation1/1 -> Sum/2

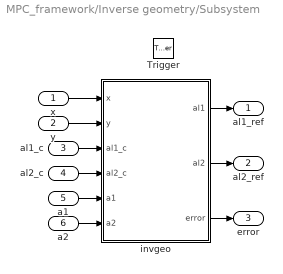
== system MPC_framework/Inverse geometry/Subsystem ==
  x : Inport
  y : Inport  Port=2
  al1_c : Inport  Port=3
  al2_c : Inport  Port=4
  a1 : Inport  Port=5
  a2 : Inport  Port=6
  Trigger : TriggerPort
  invgeo : Stateflow chart
  al1_ref : Outport
  al2_ref : Outport  Port=2
  error : Outport  Port=3
  wires:
  x/1 -> invgeo/1(x)
  y/1 -> invgeo/2(y)
  invgeo/1(al1) -> al1_ref/1
  al1_c/1 -> invgeo/3(al1_c)
  invgeo/2(al2) -> al2_ref/1
  al2_c/1 -> invgeo/4(al2_c)
  a1/1 -> invgeo/5(a1)
  invgeo/3(error) -> error/1
  a2/1 -> invgeo/6(a2)

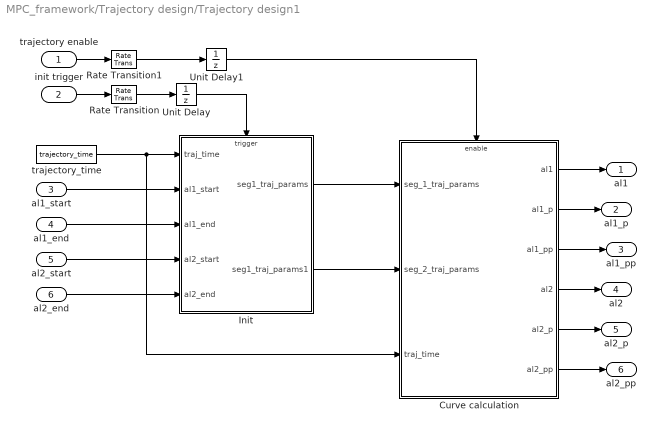
== system MPC_framework/Trajectory design/Trajectory design1 ==
  trajectory enable : Inport
  init trigger : Inport  Port=2
  al1_start : Inport  Port=3
  al1_end : Inport  Port=4
  al2_start : Inport  Port=5
  al2_end : Inport  Port=6
  Curve calculation : Subsystem
  Init : Subsystem
  Rate Transition : RateTransition  OutPortSampleTime=fundamental_sample_time
  Rate Transition1 : RateTransition  OutPortSampleTime=fundamental_sample_time
  Unit Delay : UnitDelay  SampleTime=-1
  Unit Delay1 : UnitDelay  SampleTime=-1
  trajectory_time : Constant  Value=trajectory_time  OutDataType=sfix(16)  ConRadixGroup=Use specified scaling  OutScaling=2^0  SampleTime=inf  FramePeriod=inf
  al1 : Outport
  al1_p : Outport  Port=2
  al1_pp : Outport  Port=3
  al2 : Outport  Port=4
  al2_p : Outport  Port=5
  al2_pp : Outport  Port=6
  wires:
  trajectory_time/1 -> Curve calculation/3(traj_time), Init/1(traj_time)
  al1_end/1 -> Init/3(al1_end)
  Init/2(seg1_traj_params1) -> Curve calculation/2(seg_2_traj_params)
  Init/1(seg1_traj_params) -> Curve calculation/1(seg_1_traj_params)
  trajectory enable/1 -> Rate Transition1/1
  Curve calculation/1(al1) -> al1/1
  Curve calculation/2(al1_p) -> al1_p/1
  al1_start/1 -> Init/2(al1_start)
  Curve calculation/3(al1_pp) -> al1_pp/1
  Curve calculation/4(al2) -> al2/1
  Curve calculation/5(al2_p) -> al2_p/1
  Curve calculation/6(al2_pp) -> al2_pp/1
  al2_start/1 -> Init/4(al2_start)
  al2_end/1 -> Init/5(al2_end)
  init trigger/1 -> Rate Transition/1
  Unit Delay/1 -> Init/Trigger
  Unit Delay1/1 -> Curve calculation/Enable
  Rate Transition/1 -> Unit Delay/1
  Rate Transition1/1 -> Unit Delay1/1

== system MPC_framework/async_request receiver1/async_request message unpacking ==
  note: Add any blocks to this subsystem that need to be
      | executed each time a message is received.
  Msg : Inport
  f : TriggerPort  TriggerType=function-call
  CAN Message Unpacking (CANdb) : canblocks/CAN Message Unpacking (CANdb)/CAN Message Unpacking (CANdb)
  async_request : Outport
  wires:
  Msg/1 -> CAN Message Unpacking (CANdb)/1
  CAN Message Unpacking (CANdb)/1 -> async_request/1

== system MPC_framework/incremental_in_value receiver/incremental_in_value unpacking ==
  note: Add any blocks to this subsystem that need to be
      | executed each time a message is received.
  Msg : Inport
  f : TriggerPort  TriggerType=function-call
  CAN Message Unpacking (CANdb) : canblocks/CAN Message Unpacking (CANdb)/CAN Message Unpacking (CANdb)
  cntr1 : Outport
  cntr2 : Outport  Port=2
  wires:
  Msg/1 -> CAN Message Unpacking (CANdb)/1
  CAN Message Unpacking (CANdb)/2 -> cntr2/1
  CAN Message Unpacking (CANdb)/1 -> cntr1/1

== system MPC_framework/init_ack_messages receiver/CAN Message Unpacking (CANdb) ==
  Msg : Inport
  f : TriggerPort  TriggerType=function-call
  CAN Message Unpacking (CANdb) : canblocks/CAN Message Unpacking (CANdb)/CAN Message Unpacking (CANdb)
  Compare To Constant : simulink/Logic and Bit Operations/Compare To Constant  SystemSampleTime=-1  relop===  const=init_ack_sync_message  LogicOutDataTypeMode=uint8  ZeroCross=off
  init_ack_sync received : Outport
  wires:
  Msg/1 -> CAN Message Unpacking (CANdb)/1
  CAN Message Unpacking (CANdb)/1 -> Compare To Constant/1
  Compare To Constant/1 -> init_ack_sync received/1

== system MPC_framework/init_ack_messages receiver/CAN Message Unpacking (CANdb)1 ==
  Msg : Inport
  f : TriggerPort  TriggerType=function-call
  CAN Message Unpacking (CANdb) : canblocks/CAN Message Unpacking (CANdb)/CAN Message Unpacking (CANdb)
  Compare To Constant : simulink/Logic and Bit Operations/Compare To Constant  SystemSampleTime=-1  relop===  const=init_ack_async_message  LogicOutDataTypeMode=uint8  ZeroCross=off
  init_ack_async received : Outport
  wires:
  Compare To Constant/1 -> init_ack_async received/1
  CAN Message Unpacking (CANdb)/1 -> Compare To Constant/1
  Msg/1 -> CAN Message Unpacking (CANdb)/1

== system MPC_framework/input_coords receiver/input_coords message unpacking ==
  note: Add any blocks to this subsystem that need to be
      | executed each time a message is received.
  Msg : Inport
  f : TriggerPort  TriggerType=function-call
  CAN Message Unpacking (CANdb) : canblocks/CAN Message Unpacking (CANdb)/CAN Message Unpacking (CANdb)
  x : Outport
  y : Outport  Port=2
  wires:
  Msg/1 -> CAN Message Unpacking (CANdb)/1
  CAN Message Unpacking (CANdb)/1 -> y/1
  CAN Message Unpacking (CANdb)/2 -> x/1

== system MPC_framework/operation_mode handler/operation_mode_changed sender ==
  operation_mode : Inport
  Trigger : TriggerPort
  TouCAN Transmit : mpc555toucan/TouCAN Transmit  SystemSampleTime=-1  module=A  tx_mode=Queued transmission with shared buffer  fifo_queue_length=8  bufferids=0  buffers_used=0, 1, 2  t=-1  enablePassThru=off
  operation_mode_changed message packing : canblocks/CAN Message Packing (CANdb)
  wires:
  operation_mode_changed message packing/1 -> TouCAN Transmit/1
  operation_mode/1 -> operation_mode_changed message packing/1

== system MPC_framework/primitive_button receiver/primitive_button message unpacking ==
  note: Add any blocks to this subsystem that need to be
      | executed each time a message is received.
  Msg : Inport
  f : TriggerPort  TriggerType=function-call
  CAN Message Unpacking (CANdb) : canblocks/CAN Message Unpacking (CANdb)/CAN Message Unpacking (CANdb)
  "primitive_button " : Outport
  wires:
  CAN Message Unpacking (CANdb)/1 -> "primitive_button "/1
  Msg/1 -> CAN Message Unpacking (CANdb)/1

== system MPC_framework/stop_button receiver/stop_button message packing ==
  note: Add any blocks to this subsystem that need to be
      | executed each time a message is received.
  Msg : Inport
  f : TriggerPort  TriggerType=function-call
  CAN Message Unpacking (CANdb) : canblocks/CAN Message Unpacking (CANdb)/CAN Message Unpacking (CANdb)
  stop_button received : Outport
  wires:
  Msg/1 -> CAN Message Unpacking (CANdb)/1
  CAN Message Unpacking (CANdb)/1 -> stop_button received/1

== system MPC_framework/sync_command handler/sync_command sender ==
  sync_command : Inport
  Trigger : TriggerPort
  TouCAN Transmit : mpc555toucan/TouCAN Transmit  SystemSampleTime=-1  module=A  tx_mode=Queued transmission with shared buffer  fifo_queue_length=8  bufferids=0  buffers_used=0, 1, 2  t=-1  enablePassThru=off
  sync_command message packing : canblocks/CAN Message Packing (CANdb)
  wires:
  sync_command/1 -> sync_command message packing/1
  sync_command message packing/1 -> TouCAN Transmit/1

== system MPC_framework/Controller/Discrete PD/Discrete derivative ==
  u : Inport  OutDataType=fixdt(1,16,0)  OutScaling=[]
  Td : Inport  Port=2  OutDataType=fixdt(1,16,0)  OutScaling=[]
  T : Inport  Port=3  OutDataType=fixdt(1,16,0)  OutScaling=[]
  Divide : Product  Inputs=*/  OutDataTypeMode=single  OutScaling=2^-10  InputSameDT=on
  Product : Product  OutDataTypeMode=single  RndMeth=Zero  InputSameDT=on
  Sum : Sum  Inputs=|+-
  Unit Delay : UnitDelay  SampleTime=-1
  y : Outport  OutDataType=fixdt(1,16,0)  OutScaling=[]
  wires:
  u/1 -> Unit Delay/1, Sum/1
  Unit Delay/1 -> Sum/2
  Sum/1 -> Product/1
  Td/1 -> Product/2
  Product/1 -> Divide/1
  T/1 -> Divide/2
  Divide/1 -> y/1

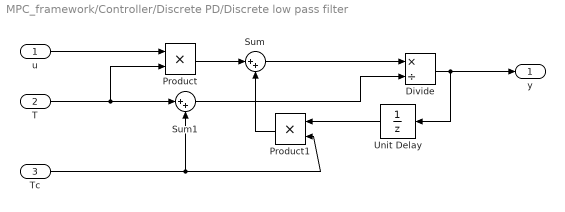
== system MPC_framework/Controller/Discrete PD/Discrete low pass filter ==
  u : Inport  OutDataType=fixdt(1,16,0)  OutScaling=[]
  T : Inport  Port=2  OutDataType=fixdt(1,16,0)  OutScaling=[]
  Tc : Inport  Port=3  OutDataType=fixdt(1,16,0)  OutScaling=[]
  Divide : Product  Inputs=*/  OutDataTypeMode=single  OutScaling=2^-10  InputSameDT=on
  Product : Product  OutDataTypeMode=single  RndMeth=Zero  InputSameDT=on
  Product1 : Product  Orientation=left  OutDataTypeMode=single  RndMeth=Zero  InputSameDT=on
  Sum : Sum  Inputs=|++
  Sum1 : Sum  Inputs=|++  OutDataTypeMode=single  InputSameDT=on
  Unit Delay : UnitDelay  Orientation=left  SampleTime=-1
  y : Outport  OutDataType=fixdt(1,16,0)  OutScaling=[]
  wires:
  u/1 -> Product/1
  T/1 -> Product/2, Sum1/1
  Unit Delay/1 -> Product1/1
  Tc/1 -> Product1/2, Sum1/2
  Product/1 -> Sum/1
  Product1/1 -> Sum/2
  Sum/1 -> Divide/1
  Sum1/1 -> Divide/2
  Divide/1 -> Unit Delay/1, y/1

== system MPC_framework/Controller/Discrete PD1/Discrete derivative ==
  u : Inport  OutDataType=fixdt(1,16,0)  OutScaling=[]
  Td : Inport  Port=2  OutDataType=fixdt(1,16,0)  OutScaling=[]
  T : Inport  Port=3  OutDataType=fixdt(1,16,0)  OutScaling=[]
  Divide : Product  Inputs=*/  OutDataTypeMode=single  OutScaling=2^-10  InputSameDT=on
  Product : Product  OutDataTypeMode=single  RndMeth=Zero  InputSameDT=on
  Sum : Sum  Inputs=|+-
  Unit Delay : UnitDelay  SampleTime=-1
  y : Outport  OutDataType=fixdt(1,16,0)  OutScaling=[]
  wires:
  u/1 -> Unit Delay/1, Sum/1
  Unit Delay/1 -> Sum/2
  Sum/1 -> Product/1
  Td/1 -> Product/2
  Product/1 -> Divide/1
  T/1 -> Divide/2
  Divide/1 -> y/1

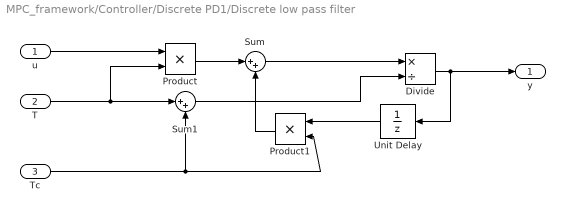
== system MPC_framework/Controller/Discrete PD1/Discrete low pass filter ==
  u : Inport  OutDataType=fixdt(1,16,0)  OutScaling=[]
  T : Inport  Port=2  OutDataType=fixdt(1,16,0)  OutScaling=[]
  Tc : Inport  Port=3  OutDataType=fixdt(1,16,0)  OutScaling=[]
  Divide : Product  Inputs=*/  OutDataTypeMode=single  OutScaling=2^-10  InputSameDT=on
  Product : Product  OutDataTypeMode=single  RndMeth=Zero  InputSameDT=on
  Product1 : Product  Orientation=left  OutDataTypeMode=single  RndMeth=Zero  InputSameDT=on
  Sum : Sum  Inputs=|++
  Sum1 : Sum  Inputs=|++  OutDataTypeMode=single  InputSameDT=on
  Unit Delay : UnitDelay  Orientation=left  SampleTime=-1
  y : Outport  OutDataType=fixdt(1,16,0)  OutScaling=[]
  wires:
  u/1 -> Product/1
  T/1 -> Product/2, Sum1/1
  Unit Delay/1 -> Product1/1
  Tc/1 -> Product1/2, Sum1/2
  Product/1 -> Sum/1
  Product1/1 -> Sum/2
  Sum/1 -> Divide/1
  Sum1/1 -> Divide/2
  Divide/1 -> Unit Delay/1, y/1

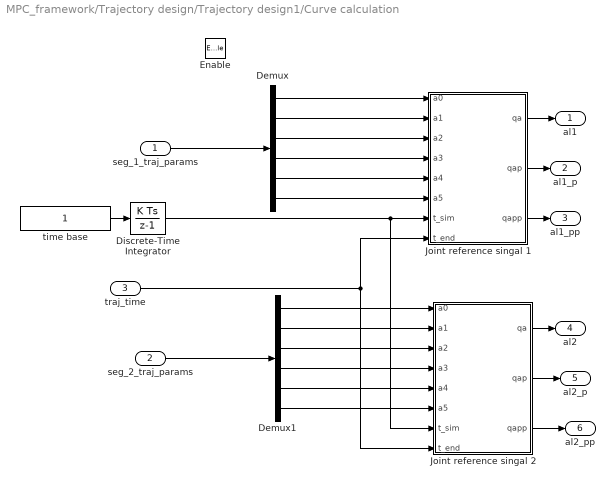
== system MPC_framework/Trajectory design/Trajectory design1/Curve calculation ==
  seg_1_traj_params : Inport
  seg_2_traj_params : Inport  Port=2
  traj_time : Inport  Port=3
  Enable : EnablePort  StatesWhenEnabling=reset
  Demux : Demux  Outputs=6
  Demux1 : Demux  Outputs=6
  Discrete-Time Integrator : DiscreteIntegrator  SampleTime=-1  ICPrevOutput=DiscIntNeverNeededParam  ICPrevScaledInput=DiscIntNeverNeededParam
  Joint reference singal 1 : Stateflow chart  TreatAsAtomicUnit=on
  Joint reference singal 2 : Stateflow chart  TreatAsAtomicUnit=on
  time base : Constant  Value=1  OutDataType=sfix(16)  ConRadixGroup=Use specified scaling  OutScaling=2^0  SampleTime=inf  FramePeriod=inf
  al1 : Outport
  al1_p : Outport  Port=2
  al1_pp : Outport  Port=3
  al2 : Outport  Port=4
  al2_p : Outport  Port=5
  al2_pp : Outport  Port=6
  wires:
  Joint reference singal 1/1(qa) -> al1/1
  Joint reference singal 1/2(qap) -> al1_p/1
  Joint reference singal 1/3(qapp) -> al1_pp/1
  Joint reference singal 2/1(qa) -> al2/1
  Discrete-Time Integrator/1 -> Joint reference singal 1/7(t_sim), Joint reference singal 2/7(t_sim)
  time base/1 -> Discrete-Time Integrator/1
  Demux/1 -> Joint reference singal 1/1(a0)
  Demux/2 -> Joint reference singal 1/2(a1)
  Demux/3 -> Joint reference singal 1/3(a2)
  Demux/4 -> Joint reference singal 1/4(a3)
  Demux/5 -> Joint reference singal 1/5(a4)
  Demux/6 -> Joint reference singal 1/6(a5)
  Demux1/1 -> Joint reference singal 2/1(a0)
  Demux1/2 -> Joint reference singal 2/2(a1)
  Demux1/3 -> Joint reference singal 2/3(a2)
  Demux1/4 -> Joint reference singal 2/4(a3)
  Demux1/5 -> Joint reference singal 2/5(a4)
  Demux1/6 -> Joint reference singal 2/6(a5)
  seg_1_traj_params/1 -> Demux/1
  seg_2_traj_params/1 -> Demux1/1
  traj_time/1 -> Joint reference singal 1/8(t_end), Joint reference singal 2/8(t_end)
  Joint reference singal 2/2(qap) -> al2_p/1
  Joint reference singal 2/3(qapp) -> al2_pp/1

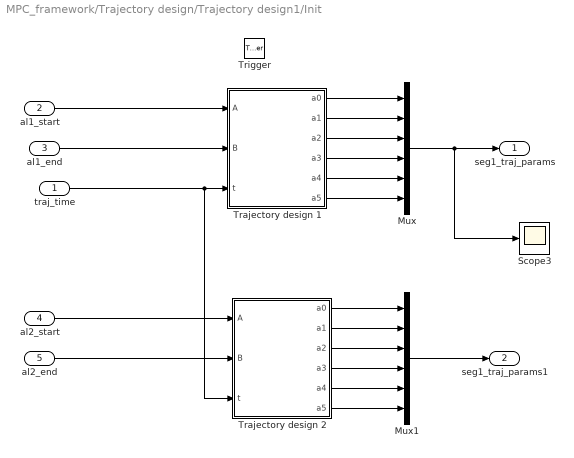
== system MPC_framework/Trajectory design/Trajectory design1/Init ==
  traj_time : Inport
  al1_start : Inport  Port=2
  al1_end : Inport  Port=3
  al2_start : Inport  Port=4
  al2_end : Inport  Port=5
  Trigger : TriggerPort
  Mux : Mux  Inputs=6
  Mux1 : Mux  Inputs=6
  Scope3 : Scope
      settings: YMin=38  YMax=42  SaveName=ScopeData5
  Trajectory design 1 : Stateflow chart  TreatAsAtomicUnit=on
  Trajectory design 2 : Stateflow chart  TreatAsAtomicUnit=on
  seg1_traj_params : Outport
  seg1_traj_params1 : Outport  Port=2
  wires:
  al1_start/1 -> Trajectory design 1/1(A)
  al1_end/1 -> Trajectory design 1/2(B)
  al2_start/1 -> Trajectory design 2/1(A)
  al2_end/1 -> Trajectory design 2/2(B)
  traj_time/1 -> Trajectory design 1/3(t), Trajectory design 2/3(t)
  Trajectory design 1/1(a0) -> Mux/1
  Trajectory design 1/2(a1) -> Mux/2
  Trajectory design 1/3(a2) -> Mux/3
  Trajectory design 1/4(a3) -> Mux/4
  Trajectory design 1/5(a4) -> Mux/5
  Trajectory design 1/6(a5) -> Mux/6
  Trajectory design 2/1(a0) -> Mux1/1
  Trajectory design 2/2(a1) -> Mux1/2
  Trajectory design 2/3(a2) -> Mux1/3
  Trajectory design 2/4(a3) -> Mux1/4
  Trajectory design 2/5(a4) -> Mux1/5
  Trajectory design 2/6(a5) -> Mux1/6
  Mux/1 -> seg1_traj_params/1, Scope3/1
  Mux1/1 -> seg1_traj_params1/1
